simulink model "BBBCSystem_IT2-FPID"  (R2023b)
settings: Solver=ode3  StartTime=0.0  StopTime=25  FixedStep=0.01  RelTol=1e-3  EnableMultiTasking=on
values from neighbouring files (symbols this model uses):
  K0 = x(i,3)    [BCostPD.m]    (also in dataset.mat = 0.0001; initiateVars.m = 0.0001; system_workspace.mat = 0.0001; system_workspace_ayk.mat = 0.0001)
  K1 = x(i,4)    [BCostPD.m]    (also in dataset.mat = 0.1; initiateVars.m = 0.1; system_workspace.mat = 0.1; system_workspace_ayk.mat = 0.1)
  Kd = x(i,2)    [BCostPD.m]    (also in dataset.mat = 2; initiateVars.m = 2; system_workspace.mat = 2; system_workspace_ayk.mat = 2)
  Ke = x(i,1)    [BCostPD.m]    (also in dataset.mat = 1; initiateVars.m = 1; system_workspace.mat = 1; system_workspace_ayk.mat = 1)
undefined symbols (not defined in the file or in its folder): DiscIntNeverNeededParam, magnitude
libraries: simulink x2, fuzblock x1
settings Model: Creator=fd  LastModifiedBy=fethi
settings SolverCC: AlgebraicLoopSolver=TrustRegion
settings DataIOCC: LimitDataPoints=on  SaveFormat=Array  SignalLoggingSaveFormat=ModelDataLogs  ReturnWorkspaceOutputs=off
settings OptimizationCC: ExpressionDepthLimit=2147483647  LifeSpan=inf
settings DebuggingCC: UnderspecifiedInitializationDetection=Classic  MergeDetectMultiDrivingBlocksExec=none  SolverPrmCheckMsg=warning  MultiTaskDSMMsg=warning  MultiTaskCondExecSysMsg=none  FcnCallInpInsideContextMsg=warning  UnconnectedInputMsg=warning  UnconnectedOutputMsg=warning  UnconnectedLineMsg=warning  StateNameClashWarn=warning  SFUnexpectedBacktrackingDiag=warning  SFNoUnconditionalDefaultTransitionDiag=warning  SFExecutionAtInitializationDiag=none  ArithmeticOperatorsInVariantConditions=warning
settings HardwareCC: ProdBitPerPointer=32  ProdBitPerSizeT=32  ProdBitPerPtrDiffT=32  ProdLargestAtomicFloat=None  ProdIntDivRoundTo=Undefined  ProdEndianess=Unspecified  ProdWordSize=32  ProdHWDeviceType=32-bit Generic
settings ModelReferenceCC: PropagateSignalLabelsOutOfModel=off
settings SFSimCC: SimUseLocalCustomCode=off  CustomCodeUndefinedFunction=UseInterfaceOnly
settings RTWCC: RTWUseLocalCustomCode=off
settings CodeAppCC: StateflowObjectComments=on
settings GRTTargetCC: TargetLangStandard=C89/C90 (ANSI)  CombineOutputUpdateFcns=off  GRTInterface=on
settings ConfigComp: CovMetricSettings=dw  CovSaveCumulativeToWorkspaceVar=on  CovSaveSingleToWorkspaceVar=on  CovExternalEMLEnable=off

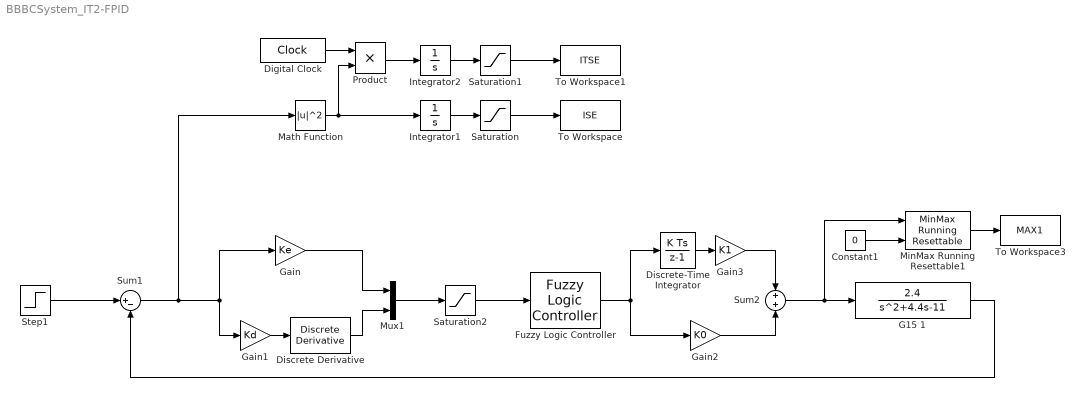
== system BBBCSystem_IT2-FPID ==
  Constant1 : Constant  Value=0
  Digital Clock : DigitalClock  SampleTime=0.01
  Discrete Derivative : simulink/Discrete/Discrete Derivative  gainval=1.0  ICPrevScaledInput=0.0  OutMin=[]  OutMax=[]  OutDataType=fixdt(1, 16)  OutScaling=2^-10  DoSatur=off
  Discrete-Time Integrator : DiscreteIntegrator  SampleTime=-1  ICPrevOutput=DiscIntNeverNeededParam  ICPrevScaledInput=DiscIntNeverNeededParam
  Fuzzy Logic Controller : fuzblock/Fuzzy Logic  Controller  FIS='fis2.fis'  OutputSampleNumber=101  DataType=double  FuzzifiedInputs=off  RuleFiringStrengths=off  RuleOutputs=off  AggregatedOutputs=off  SimulateUsing=Interpreted execution  OutOfRangeInputValueMessage=warning  NoRuleFiredMessage=warning  EmptyOutputFuzzySetMessage=warning
  G15 1 : TransferFcn  Numerator=[2.4]  Denominator=[1 4.4 -11]
  Gain : Gain  Gain=Ke
  Gain1 : Gain  Gain=Kd
  Gain2 : Gain  Gain=K0
  Gain3 : Gain  Gain=K1
  Integrator1 : Integrator
  Integrator2 : Integrator
  Math Function : Math  Operator=magnitude^2  SignedPower=on
  MinMax Running Resettable1 : simulink/Math Operations/MinMax Running Resettable  Function=max  vinit=0
  Mux1 : Mux  Inputs=2
  Product : Product  RndMeth=Zero
  Saturation : Saturate  UpperLimit=800
  Saturation1 : Saturate  UpperLimit=800
  Saturation2 : Saturate  UpperLimit=1  LowerLimit=-1
  Step1 : Step  Time=0  SampleTime=0.01
  Sum1 : Sum  Inputs=|+-
  Sum2 : Sum  Inputs=+|+
  To Workspace : ToWorkspace  VariableName=ISE  SampleTime=-1
  To Workspace1 : ToWorkspace  VariableName=ITSE  SampleTime=-1
  To Workspace3 : ToWorkspace  VariableName=MAX1  SampleTime=-1
  wires:
  Integrator1/1 -> Saturation/1
  Math Function/1 -> Product/2, Integrator1/1
  Saturation/1 -> To Workspace/1
  Digital Clock/1 -> Product/1
  Product/1 -> Integrator2/1
  Integrator2/1 -> Saturation1/1
  Saturation1/1 -> To Workspace1/1
  Discrete Derivative/1 -> Mux1/2
  Gain3/1 -> Sum2/1
  Gain2/1 -> Sum2/2
  Gain1/1 -> Discrete Derivative/1
  Fuzzy Logic Controller/1 -> Gain2/1, Discrete-Time Integrator/1
  Discrete-Time Integrator/1 -> Gain3/1
  Step1/1 -> Sum1/1
  Gain/1 -> Mux1/1
  G15 1/1 -> Sum1/2
  Constant1/1 -> MinMax Running Resettable1/2
  MinMax Running Resettable1/1 -> To Workspace3/1
  Sum2/1 -> MinMax Running Resettable1/1, G15 1/1
  Sum1/1 -> Math Function/1, Gain1/1, Gain/1
  Mux1/1 -> Saturation2/1
  Saturation2/1 -> Fuzzy Logic Controller/1
